simulink model "nonlinear_system"  (R2018a)
settings: Solver=VariableStepAuto  StartTime=0.0  StopTime=sim_params.T  RelTol=1e-3
undefined symbols (not defined in the file or in its folder): sim_params
settings Model: Creator=applicon  LastModifiedBy=applicon
settings DataIOCC: ExternalInput=[sim_params.t, sim_params.u']  InitialState=x0  LoadExternalInput=on  SaveFormat=Array  SaveState=on  SignalLogging=off  DSMLogging=off  StateSaveName=x_out  TimeSaveName=t_out  OutputSaveName=y_out

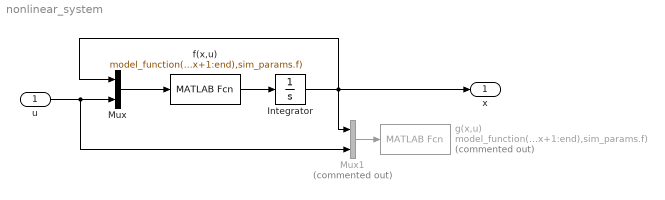
== system nonlinear_system ==
  u : Inport  PortDimensions=sim_params.nu
  Integrator : Integrator  InitialCondition=sim_params.xi
  Mux : Mux  Inputs=2
  Mux1 : Mux  Commented=on  Inputs=2
  f(x,u) : MATLABFcn  MATLABFcn=model_function(u(1:sim_params.nx),u(sim_params.nx+1:end),sim_params.f)
  g(x,u) : MATLABFcn  Commented=on  MATLABFcn=model_function(u(1:sim_params.nx),u(sim_params.nx+1:end),sim_params.f)
  x : Outport  PortDimensions=sim_params.ny
  wires:
  Mux/1 -> f(x,u)/1
  u/1 -> Mux1/2, Mux/2
  f(x,u)/1 -> Integrator/1
  Integrator/1 -> Mux1/1, x/1, Mux/1
  Mux1/1 -> g(x,u)/1
